simulink model "CSEV"  (R2022b)
settings: Solver=FixedStepDiscrete  StartTime=0.0  StopTime=50000000  FixedStep=1  RelTol=1e-3
libraries: simulink x20
settings Model: Creator=sadamu  LastModifiedBy=程一帆
settings OptimizationCC: DefaultParameterBehavior=Inlined  BufferReuse=off  GlobalBufferReuse=off  ExpressionFolding=off  EnableMemcpy=off  PassReuseOutputArgsAs=Individual arguments  NoFixptDivByZeroProtection=on  EfficientFloat2IntCast=on  OptimizeDataStoreBuffers=off  BusAssignmentInplaceUpdate=off  OptimizationLevel=level0  EfficientTunableParamExpr=on
settings DebuggingCC: ParameterDowncastMsg=warning  ParameterTunabilityLossMsg=error
settings SFSimCC: MATLABDynamicMemAlloc=off
settings RTWCC: Description=Embedded Coder  SystemTargetFile=ert.tlc  GenCodeOnly=on  TemplateMakefile=ert_default_tmf
settings CodeAppCC: ForceParamTrailComments=on  IgnoreCustomStorageClasses=off  OperatorAnnotations=on  SimulinkDataObjDesc=on  SFDataObjDesc=on  InsertBlockDesc=on
settings ERTTargetCC: TargetLangStandard=C99 (ISO)  GenerateSampleERTMain=on  CodeInterfacePackaging=Reusable function  InlinedParameterPlacement=NonHierarchical  ERTCustomFileTemplate=example_file_process.tlc
settings ConfigComp: CovMetricSettings=dcmwe  DVMaxProcessTime=3600  DVTestSuiteOptimization=Auto  DVDetectOutOfBounds=on  DVModelReferenceHarness=on

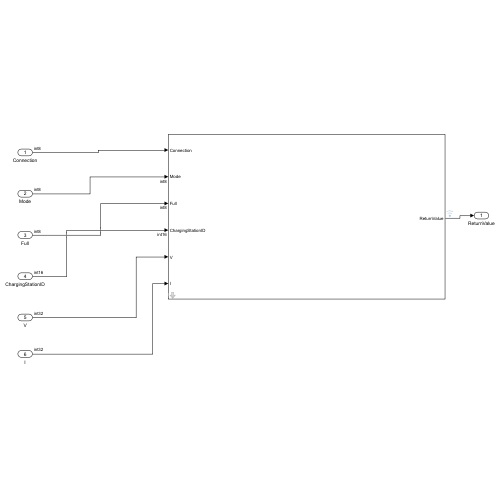
[thumbnail: Simulink's stored preview of the top-level diagram]
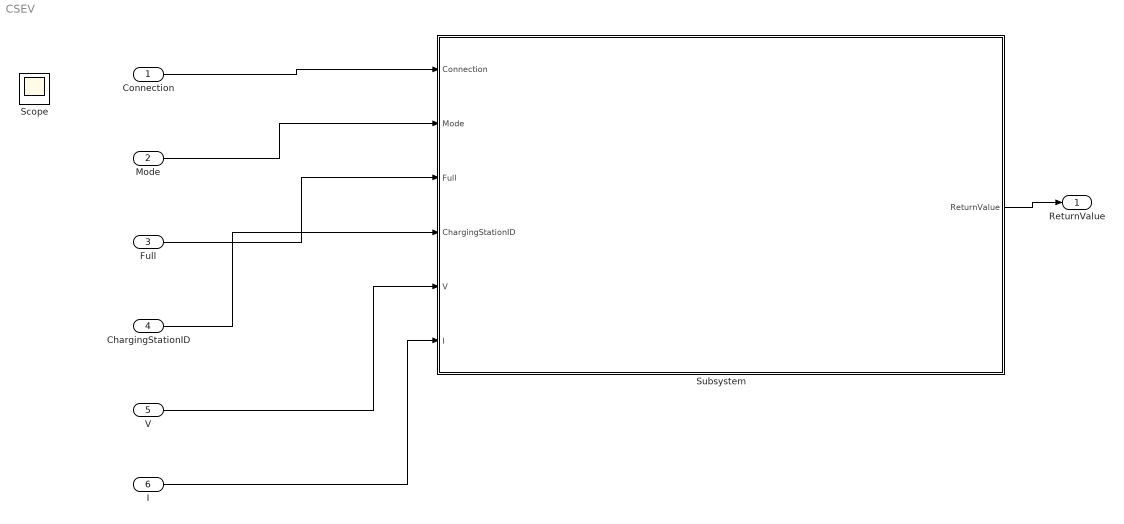
== system CSEV ==
  Connection : Inport  OutDataTypeStr=int8
  Mode : Inport  Port=2  OutDataTypeStr=int8
  Full : Inport  Port=3  OutDataTypeStr=int8
  ChargingStationID : Inport  Port=4  OutDataTypeStr=int16
  V : Inport  Port=5  OutDataTypeStr=int32
  I : Inport  Port=6  OutDataTypeStr=int32
  Subsystem : Subsystem  mask{Len=16}
      mask DialogControl ParameterGroupVar Prompt: 参数
  ReturnValue : Outport
  Scope : Scope
  wires:
  Connection/1 -> Subsystem/1(Connection)
  Mode/1 -> Subsystem/2(Mode)
  Full/1 -> Subsystem/3(Full)
  ChargingStationID/1 -> Subsystem/4(ChargingStationID)
  Subsystem/1(ReturnValue) -> ReturnValue/1
  V/1 -> Subsystem/5(V)
  I/1 -> Subsystem/6(I)

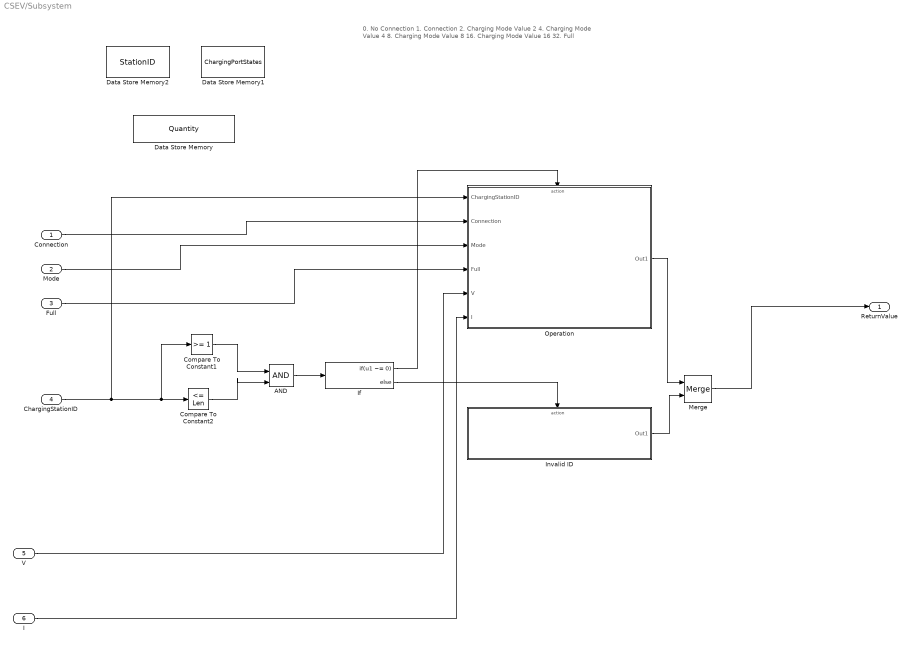
== system CSEV/Subsystem ==
  note: 0. No Connection
      | 1. Connection
      | 2. Charging Mode Value 2
      | 4. Charging Mode Value 4
      | 8. Charging Mode Value 8
      | 16. Charging Mode Value 16
      | 32. Full
  Connection : Inport
  Mode : Inport  Port=2  OutDataTypeStr=int8
  Full : Inport  Port=3  OutDataTypeStr=int8
  ChargingStationID : Inport  Port=4  OutDataTypeStr=int16
  V : Inport  Port=5
  I : Inport  Port=6
  AND : Logic  IconShape=distinctive  AllPortsSameDT=off  OutDataTypeStr=boolean
  Compare To Constant1 : simulink/Logic and Bit Operations/Compare To Constant  relop=>=  const=1  OutDataTypeStr=boolean
  Compare To Constant2 : simulink/Logic and Bit Operations/Compare To Constant  relop=<=  const=Len  OutDataTypeStr=boolean
  Data Store Memory : DataStoreMemory  DataStoreName=Quantity  WriteAfterWriteMsg=warning  ShowAdditionalParam=off  OutDataTypeStr=int64
  Data Store Memory1 : DataStoreMemory  DataStoreName=ChargingPortStates  WriteAfterWriteMsg=warning  ShowAdditionalParam=off  OutDataTypeStr=int32  Dimensions=Len
  Data Store Memory2 : DataStoreMemory  DataStoreName=StationID  WriteAfterWriteMsg=warning  ShowAdditionalParam=off  OutDataTypeStr=int32  Dimensions=Len
  If : If  IfExpression=u1 ~= 0
  Invalid ID : Subsystem  TreatAsAtomicUnit=on
  Merge : Merge
  Operation : Subsystem  TreatAsAtomicUnit=on
  ReturnValue : Outport
  wires:
  Connection/1 -> Operation/2(Connection)
  ChargingStationID/1 -> Operation/1(ChargingStationID), Compare To Constant2/1, Compare To Constant1/1
  Compare To Constant1/1 -> AND/1
  Compare To Constant2/1 -> AND/2
  AND/1 -> If/1
  If/2 -> Invalid ID/Action
  Invalid ID/1(Out1) -> Merge/2
  Merge/1 -> ReturnValue/1
  If/1 -> Operation/Action
  Operation/1(Out1) -> Merge/1
  Mode/1 -> Operation/3(Mode)
  Full/1 -> Operation/4(Full)
  V/1 -> Operation/5(V)
  I/1 -> Operation/6(I)

== system CSEV/Subsystem/Invalid ID ==
  Action Port : ActionPort  ActionPortLabel=else
  Constant : Constant  Value=-1  OutDataTypeStr=int32
  Out1 : Outport
  wires:
  Constant/1 -> Out1/1

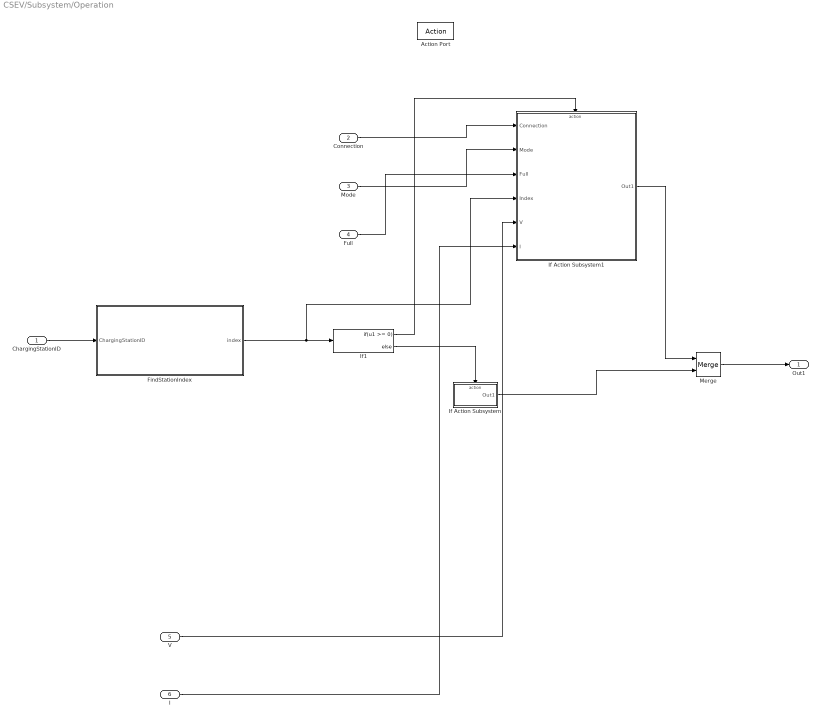
== system CSEV/Subsystem/Operation ==
  ChargingStationID : Inport  OutDataTypeStr=int16
  Connection : Inport  Port=2
  Mode : Inport  Port=3
  Full : Inport  Port=4
  V : Inport  Port=5
  I : Inport  Port=6
  Action Port : ActionPort  ActionPortLabel=if(u1 ~= 0)
  FindStationIndex : Subsystem  TreatAsAtomicUnit=on
  If Action Subsystem : Subsystem  TreatAsAtomicUnit=on
  If Action Subsystem1 : Subsystem  TreatAsAtomicUnit=on
  If1 : If  IfExpression=u1 >= 0
  Merge : Merge
  Out1 : Outport
  wires:
  ChargingStationID/1 -> FindStationIndex/1(ChargingStationID)
  FindStationIndex/1(index) -> If Action Subsystem1/4(Index), If1/1
  If1/2 -> If Action Subsystem/Action
  If1/1 -> If Action Subsystem1/Action
  If Action Subsystem1/1(Out1) -> Merge/1
  If Action Subsystem/1(Out1) -> Merge/2
  Merge/1 -> Out1/1
  Mode/1 -> If Action Subsystem1/2(Mode)
  Connection/1 -> If Action Subsystem1/1(Connection)
  Full/1 -> If Action Subsystem1/3(Full)
  V/1 -> If Action Subsystem1/5(V)
  I/1 -> If Action Subsystem1/6(I)

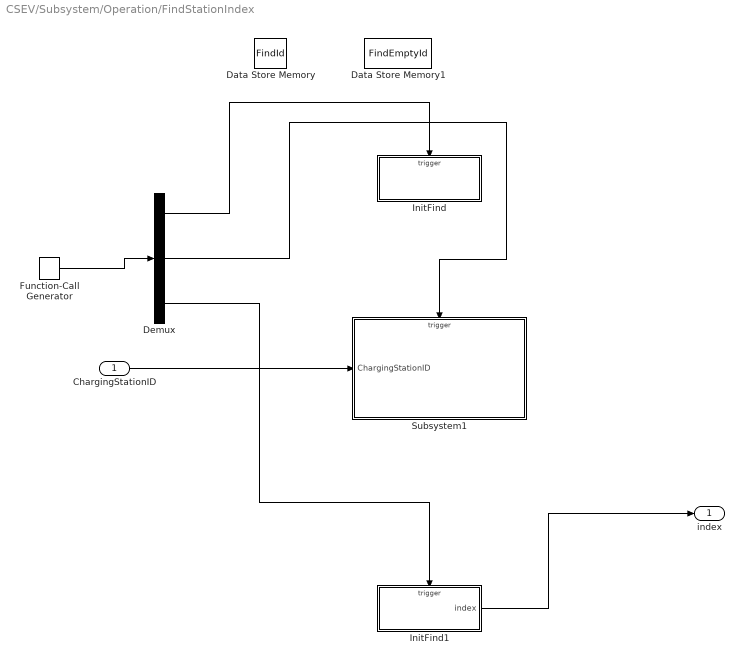
== system CSEV/Subsystem/Operation/FindStationIndex ==
  ChargingStationID : Inport
  Data Store Memory : DataStoreMemory  DataStoreName=FindId  WriteAfterWriteMsg=warning  ShowAdditionalParam=off  OutDataTypeStr=int16
  Data Store Memory1 : DataStoreMemory  DataStoreName=FindEmptyId  WriteAfterWriteMsg=warning  ShowAdditionalParam=off  OutDataTypeStr=int16
  Demux : Demux  Outputs=3
  Function-Call Generator : simulink/Ports & Subsystems/Function-Call Generator  sample_time=1  numberOfIterations=1  DisallowWideOutput=off
  InitFind : Subsystem
  InitFind1 : Subsystem
  Subsystem1 : Subsystem
  index : Outport
  wires:
  Function-Call Generator/1 -> Demux/1
  Demux/1 -> InitFind/Trigger
  Demux/2 -> Subsystem1/Trigger
  ChargingStationID/1 -> Subsystem1/1(ChargingStationID)
  InitFind1/1(index) -> index/1
  Demux/3 -> InitFind1/Trigger

== system CSEV/Subsystem/Operation/If Action Subsystem ==
  Action Port : ActionPort  ActionPortLabel=else
  Constant : Constant  Value=-2  OutDataTypeStr=int32
  Out1 : Outport
  wires:
  Constant/1 -> Out1/1

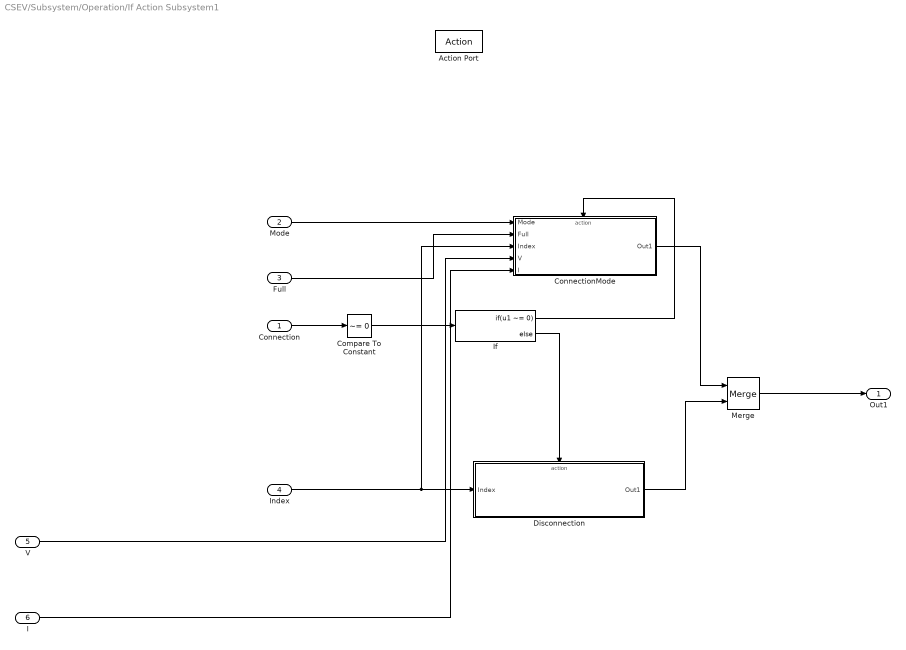
== system CSEV/Subsystem/Operation/If Action Subsystem1 ==
  Connection : Inport
  Mode : Inport  Port=2
  Full : Inport  Port=3
  Index : Inport  Port=4  OutDataTypeStr=int16
  V : Inport  Port=5
  I : Inport  Port=6
  Action Port : ActionPort  ActionPortLabel=if(u1 >= 0)
  Compare To Constant : simulink/Logic and Bit Operations/Compare To Constant  relop=~=  const=0  OutDataTypeStr=boolean
  ConnectionMode : Subsystem  TreatAsAtomicUnit=on
  Disconnection : Subsystem  TreatAsAtomicUnit=on
  If : If  IfExpression=u1 ~= 0
  Merge : Merge
  Out1 : Outport
  wires:
  Mode/1 -> ConnectionMode/1(Mode)
  Index/1 -> ConnectionMode/3(Index), Disconnection/1(Index)
  Compare To Constant/1 -> If/1
  If/2 -> Disconnection/Action
  Full/1 -> ConnectionMode/2(Full)
  Connection/1 -> Compare To Constant/1
  If/1 -> ConnectionMode/Action
  ConnectionMode/1(Out1) -> Merge/1
  Disconnection/1(Out1) -> Merge/2
  Merge/1 -> Out1/1
  V/1 -> ConnectionMode/4(V)
  I/1 -> ConnectionMode/5(I)

== system CSEV/Subsystem/Operation/FindStationIndex/InitFind ==
  function : TriggerPort  TriggerType=function-call  VariantControl=Variant
  Constant : Constant  Value=-1  OutDataTypeStr=int16
  Constant1 : Constant  Value=-1  OutDataTypeStr=int16
  Data Store Write : DataStoreWrite  DataStoreName=FindEmptyId  IndexOptions=Index vector (dialog)  Indices=1  OutputSizes=1
  Data Store Write1 : DataStoreWrite  DataStoreName=FindId  IndexOptions=Index vector (dialog)  Indices=1  OutputSizes=1
  wires:
  Constant/1 -> Data Store Write1/1
  Constant1/1 -> Data Store Write/1

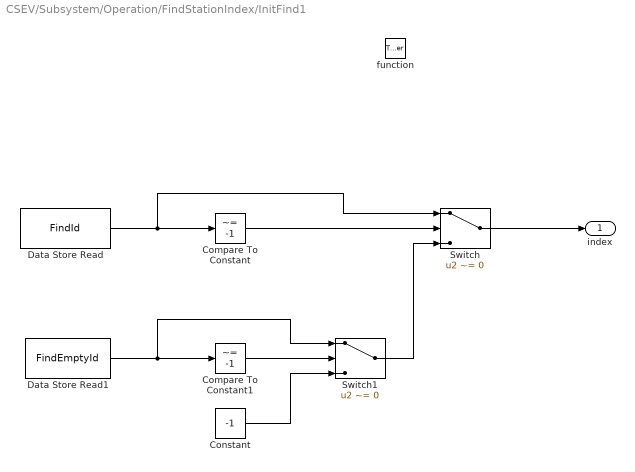
== system CSEV/Subsystem/Operation/FindStationIndex/InitFind1 ==
  function : TriggerPort  TriggerType=function-call  VariantControl=Variant
  Compare To Constant : simulink/Logic and Bit Operations/Compare To Constant  relop=~=  const=-1  OutDataTypeStr=boolean
  Compare To Constant1 : simulink/Logic and Bit Operations/Compare To Constant  relop=~=  const=-1  OutDataTypeStr=boolean
  Constant : Constant  Value=-1  OutDataTypeStr=int16
  Data Store Read : DataStoreRead  DataStoreName=FindId  IndexOptions=Index vector (dialog)  Indices=1  OutputSizes=1
  Data Store Read1 : DataStoreRead  DataStoreName=FindEmptyId  IndexOptions=Index vector (dialog)  Indices=1  OutputSizes=1
  Switch : Switch  Criteria=u2 ~= 0  SaturateOnIntegerOverflow=off  InputSameDT=off
  Switch1 : Switch  Criteria=u2 ~= 0  SaturateOnIntegerOverflow=off  InputSameDT=off
  index : Outport
  wires:
  Data Store Read/1 -> Switch/1, Compare To Constant/1
  Compare To Constant/1 -> Switch/2
  Data Store Read1/1 -> Switch1/1, Compare To Constant1/1
  Compare To Constant1/1 -> Switch1/2
  Switch1/1 -> Switch/3
  Constant/1 -> Switch1/3
  Switch/1 -> index/1

== system CSEV/Subsystem/Operation/FindStationIndex/Subsystem1 ==
  ChargingStationID : Inport
  function : TriggerPort  TriggerType=function-call  VariantControl=Variant
  Subsystem : Subsystem
  wires:
  ChargingStationID/1 -> Subsystem/1(ChargingStationID)

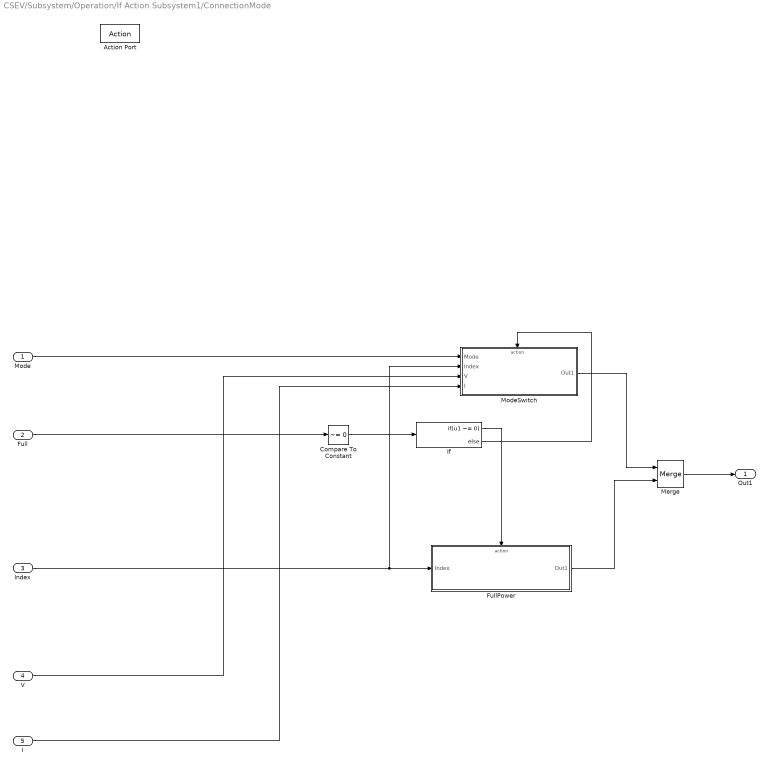
== system CSEV/Subsystem/Operation/If Action Subsystem1/ConnectionMode ==
  Mode : Inport
  Full : Inport  Port=2
  Index : Inport  Port=3  OutDataTypeStr=int16
  V : Inport  Port=4
  I : Inport  Port=5
  Action Port : ActionPort  ActionPortLabel=if(u1 ~= 0)
  Compare To Constant : simulink/Logic and Bit Operations/Compare To Constant  relop=~=  const=0  OutDataTypeStr=boolean
  FullPower : Subsystem  TreatAsAtomicUnit=on
  If : If  IfExpression=u1 ~= 0
  Merge : Merge
  ModeSwitch : Subsystem  TreatAsAtomicUnit=on
  Out1 : Outport
  wires:
  Index/1 -> ModeSwitch/2(Index), FullPower/1(Index)
  Mode/1 -> ModeSwitch/1(Mode)
  Compare To Constant/1 -> If/1
  If/2 -> ModeSwitch/Action
  Full/1 -> Compare To Constant/1
  If/1 -> FullPower/Action
  ModeSwitch/1(Out1) -> Merge/1
  FullPower/1(Out1) -> Merge/2
  Merge/1 -> Out1/1
  V/1 -> ModeSwitch/3(V)
  I/1 -> ModeSwitch/4(I)

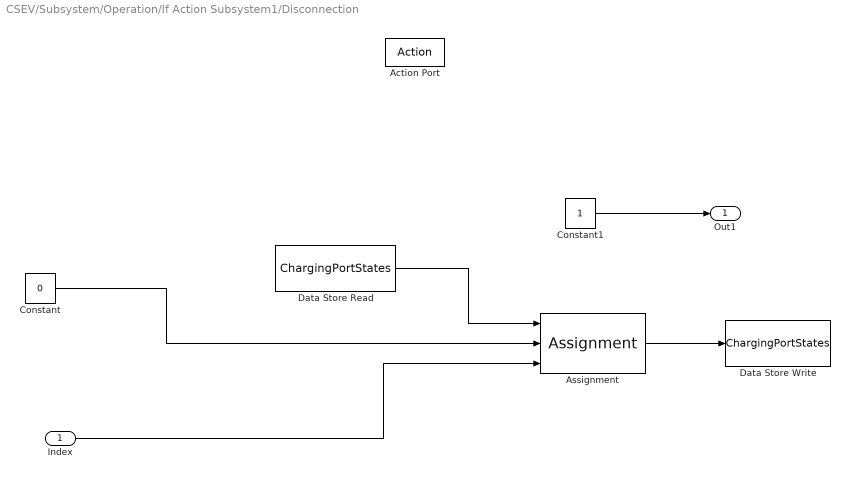
== system CSEV/Subsystem/Operation/If Action Subsystem1/Disconnection ==
  Index : Inport
  Action Port : ActionPort  ActionPortLabel=else
  Assignment : Assignment  IndexMode=Zero-based  DiagnosticForDimensions=Warning  IndexOptions=Index vector (port)  Indices=1  OutputSizes=1
  Constant : Constant  Value=0  OutDataTypeStr=int32
  Constant1 : Constant  OutDataTypeStr=int32
  Data Store Read : DataStoreRead  DataStoreName=ChargingPortStates  IndexOptions=Index vector (dialog)  Indices=1  OutputSizes=1
  Data Store Write : DataStoreWrite  DataStoreName=ChargingPortStates  IndexOptions=Index vector (dialog)  Indices=1  OutputSizes=1
  Out1 : Outport
  wires:
  Data Store Read/1 -> Assignment/1
  Assignment/1 -> Data Store Write/1
  Index/1 -> Assignment/3
  Constant/1 -> Assignment/2
  Constant1/1 -> Out1/1

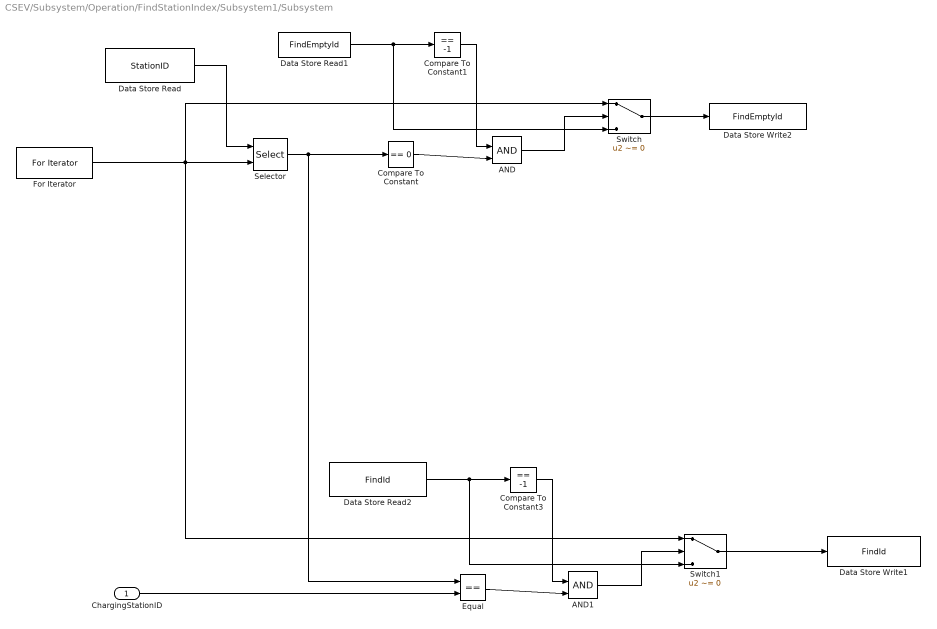
== system CSEV/Subsystem/Operation/FindStationIndex/Subsystem1/Subsystem ==
  ChargingStationID : Inport
  AND : Logic  IconShape=distinctive  AllPortsSameDT=off  OutDataTypeStr=boolean
  AND1 : Logic  IconShape=distinctive  AllPortsSameDT=off  OutDataTypeStr=boolean
  Compare To Constant : simulink/Logic and Bit Operations/Compare To Constant  relop===  const=0  OutDataTypeStr=boolean
  Compare To Constant1 : simulink/Logic and Bit Operations/Compare To Constant  relop===  const=-1  OutDataTypeStr=boolean
  Compare To Constant3 : simulink/Logic and Bit Operations/Compare To Constant  relop===  const=-1  OutDataTypeStr=boolean
  Data Store Read : DataStoreRead  DataStoreName=StationID  IndexOptions=Index vector (dialog)  Indices=1  OutputSizes=1
  Data Store Read1 : DataStoreRead  DataStoreName=FindEmptyId  IndexOptions=Index vector (dialog)  Indices=1  OutputSizes=1
  Data Store Read2 : DataStoreRead  DataStoreName=FindId  IndexOptions=Index vector (dialog)  Indices=1  OutputSizes=1
  Data Store Write1 : DataStoreWrite  DataStoreName=FindId  IndexOptions=Index vector (dialog)  Indices=1  OutputSizes=1
  Data Store Write2 : DataStoreWrite  DataStoreName=FindEmptyId  IndexOptions=Index vector (dialog)  Indices=1  OutputSizes=1
  Equal : RelationalOperator  Operator===  OutDataTypeStr=boolean  RndMeth=Simplest  InputSameDT=off
  For Iterator : ForIterator  IterationLimit=Len  IndexMode=Zero-based  IterationVariableDataType=int16
  Selector : Selector  IndexMode=Zero-based  InputPortWidth=Len  IndexOptions=Index vector (port)  Indices=[1 3]  OutputSizes=1
  Switch : Switch  Criteria=u2 ~= 0  SaturateOnIntegerOverflow=off  InputSameDT=off
  Switch1 : Switch  Criteria=u2 ~= 0  SaturateOnIntegerOverflow=off  InputSameDT=off
  wires:
  Data Store Read/1 -> Selector/1
  Selector/1 -> Equal/1, Compare To Constant/1
  Compare To Constant/1 -> AND/2
  Data Store Read1/1 -> Switch/3, Compare To Constant1/1
  Compare To Constant1/1 -> AND/1
  AND/1 -> Switch/2
  Switch/1 -> Data Store Write2/1
  Equal/1 -> AND1/2
  AND1/1 -> Switch1/2
  Compare To Constant3/1 -> AND1/1
  Data Store Read2/1 -> Switch1/3, Compare To Constant3/1
  Switch1/1 -> Data Store Write1/1
  ChargingStationID/1 -> Equal/2
  For Iterator/1 -> Switch1/1, Switch/1, Selector/2

== system CSEV/Subsystem/Operation/If Action Subsystem1/ConnectionMode/FullPower ==
  Index : Inport
  Action Port : ActionPort  ActionPortLabel=if(u1 ~= 0)
  Assignment : Assignment  IndexMode=Zero-based  DiagnosticForDimensions=Warning  IndexOptions=Index vector (port)  Indices=1  OutputSizes=1
  Constant : Constant  Value=32  OutDataTypeStr=int32
  Constant1 : Constant  OutDataTypeStr=int32
  Data Store Read : DataStoreRead  DataStoreName=ChargingPortStates  IndexOptions=Index vector (dialog)  Indices=1  OutputSizes=1
  Data Store Write : DataStoreWrite  DataStoreName=ChargingPortStates  IndexOptions=Index vector (dialog)  Indices=1  OutputSizes=1
  Out1 : Outport
  wires:
  Data Store Read/1 -> Assignment/1
  Assignment/1 -> Data Store Write/1
  Index/1 -> Assignment/3
  Constant/1 -> Assignment/2
  Constant1/1 -> Out1/1

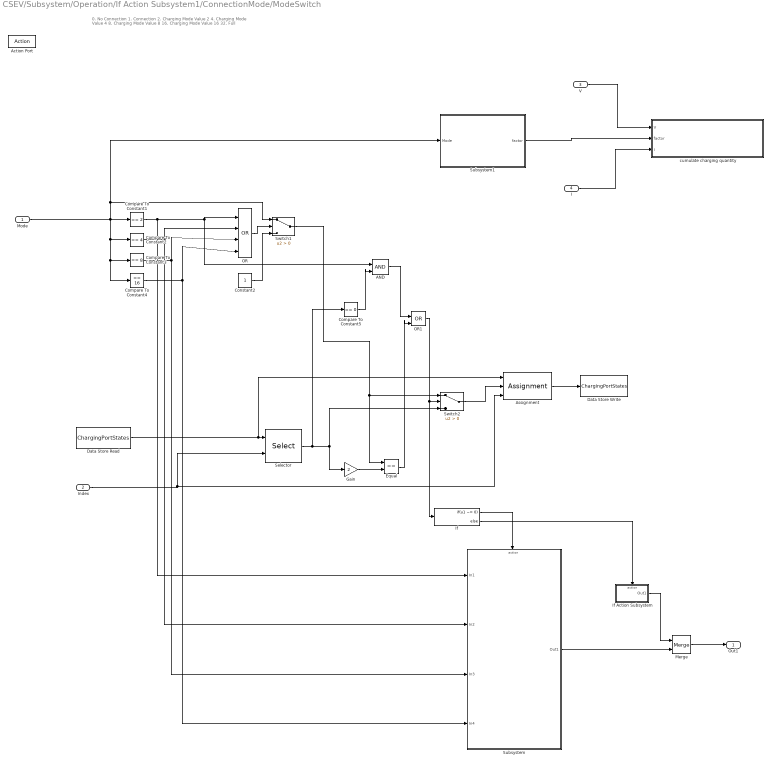
== system CSEV/Subsystem/Operation/If Action Subsystem1/ConnectionMode/ModeSwitch ==
  note: 0. No Connection
      | 1. Connection
      | 2. Charging Mode Value 2
      | 4. Charging Mode Value 4
      | 8. Charging Mode Value 8
      | 16. Charging Mode Value 16
      | 32. Full
  Mode : Inport
  Index : Inport  Port=2  OutDataTypeStr=int16
  V : Inport  Port=3
  I : Inport  Port=4
  Action Port : ActionPort  ActionPortLabel=else
  AND : Logic  IconShape=distinctive  AllPortsSameDT=off  OutDataTypeStr=boolean
  Assignment : Assignment  IndexMode=Zero-based  DiagnosticForDimensions=Warning  IndexOptions=Index vector (port)  Indices=1  OutputSizes=1
  Compare To Constant1 : simulink/Logic and Bit Operations/Compare To Constant  relop===  const=2  OutDataTypeStr=boolean
  Compare To Constant2 : simulink/Logic and Bit Operations/Compare To Constant  relop===  const=4  OutDataTypeStr=boolean
  Compare To Constant3 : simulink/Logic and Bit Operations/Compare To Constant  relop===  const=8  OutDataTypeStr=boolean
  Compare To Constant4 : simulink/Logic and Bit Operations/Compare To Constant  relop===  const=16  OutDataTypeStr=boolean
  Compare To Constant5 : simulink/Logic and Bit Operations/Compare To Constant  relop===  const=0  OutDataTypeStr=boolean
  Constant2 : Constant  OutDataTypeStr=int32
  Data Store Read : DataStoreRead  DataStoreName=ChargingPortStates  IndexOptions=Index vector (dialog)  Indices=1  OutputSizes=1
  Data Store Write : DataStoreWrite  DataStoreName=ChargingPortStates  IndexOptions=Index vector (dialog)  Indices=1  OutputSizes=1
  Equal : RelationalOperator  Operator===  OutDataTypeStr=boolean  RndMeth=Simplest  InputSameDT=off
  Gain : Gain  Gain=2  OutDataTypeStr=int32
  If : If  IfExpression=u1 ~= 0
  If Action Subsystem : Subsystem  TreatAsAtomicUnit=on
  Merge : Merge
  OR : Logic  Operator=OR  Inputs=4  IconShape=distinctive  AllPortsSameDT=off  OutDataTypeStr=boolean
  OR1 : Logic  Operator=OR  IconShape=distinctive  AllPortsSameDT=off  OutDataTypeStr=boolean
  Selector : Selector  IndexMode=Zero-based  InputPortWidth=Len  IndexOptions=Index vector (port)  Indices=[1 3]  OutputSizes=1
  Subsystem : Subsystem
  Subsystem1 : Subsystem
  Switch1 : Switch  Criteria=u2 > Threshold  SaturateOnIntegerOverflow=off  InputSameDT=off
  Switch2 : Switch  Criteria=u2 > Threshold  SaturateOnIntegerOverflow=off  InputSameDT=off
  cumulate charging quantity : Subsystem
  Out1 : Outport
  wires:
  Switch1/1 -> Equal/1, Switch2/1
  Data Store Read/1 -> Assignment/1, Selector/1
  OR/1 -> Switch1/2
  Compare To Constant3/1 -> Subsystem/3(In3), OR/3
  Compare To Constant4/1 -> Subsystem/4(In4), OR/4
  Compare To Constant1/1 -> Subsystem/1(In1), AND/1, OR/1
  Compare To Constant2/1 -> Subsystem/2(In2), OR/2
  Mode/1 -> Subsystem1/1(Mode), Switch1/1, Compare To Constant1/1, Compare To Constant4/1, Compare To Constant3/1, Compare To Constant2/1
  Constant2/1 -> Switch1/3
  Assignment/1 -> Data Store Write/1
  Index/1 -> Selector/2, Assignment/3
  Selector/1 -> Compare To Constant5/1, Gain/1, Switch2/3
  Switch2/1 -> Assignment/2
  If Action Subsystem/1(Out1) -> Merge/1
  Subsystem/1(Out1) -> Merge/2
  Merge/1 -> Out1/1
  Gain/1 -> Equal/2
  If/1 -> Subsystem/Action
  If/2 -> If Action Subsystem/Action
  Compare To Constant5/1 -> AND/2
  AND/1 -> OR1/1
  Equal/1 -> OR1/2
  OR1/1 -> If/1, Switch2/2
  V/1 -> cumulate charging quantity/1(V)
  I/1 -> cumulate charging quantity/3(I)
  Subsystem1/1(factor) -> cumulate charging quantity/2(factor)

== system CSEV/Subsystem/Operation/If Action Subsystem1/ConnectionMode/ModeSwitch/If Action Subsystem ==
  Action Port : ActionPort  ActionPortLabel=else
  Constant2 : Constant  Value=32  OutDataTypeStr=int32
  Out1 : Outport
  wires:
  Constant2/1 -> Out1/1

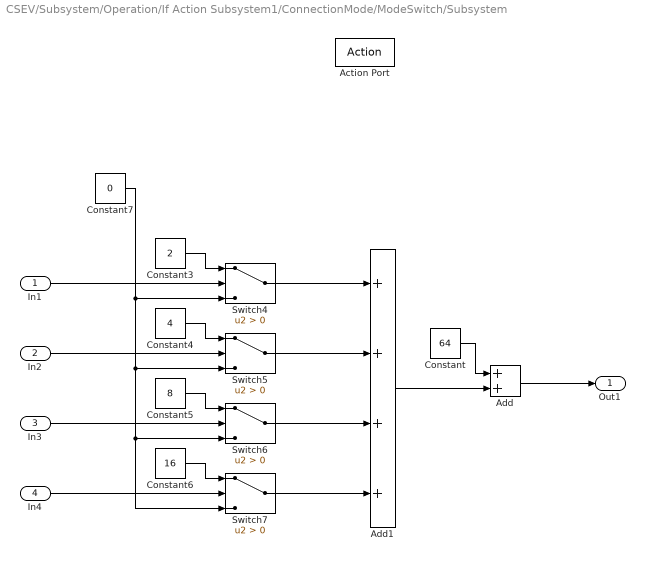
== system CSEV/Subsystem/Operation/If Action Subsystem1/ConnectionMode/ModeSwitch/Subsystem ==
  In1 : Inport
  In2 : Inport  Port=2
  In3 : Inport  Port=3
  In4 : Inport  Port=4
  Action Port : ActionPort  ActionPortLabel=if(u1 ~= 0)
  Add : Sum
  Add1 : Sum  Inputs=++++
  Constant : Constant  Value=64  OutDataTypeStr=int32
  Constant3 : Constant  Value=2  OutDataTypeStr=int32
  Constant4 : Constant  Value=4  OutDataTypeStr=int32
  Constant5 : Constant  Value=8  OutDataTypeStr=int32
  Constant6 : Constant  Value=16  OutDataTypeStr=int32
  Constant7 : Constant  Value=0  OutDataTypeStr=int32
  Switch{4..7} (4 alike) : Switch  Criteria=u2 > Threshold  SaturateOnIntegerOverflow=off  InputSameDT=off
  Out1 : Outport
  wires:
  Constant6/1 -> Switch7/1
  In1/1 -> Switch4/2
  Switch5/1 -> Add1/2
  Add1/1 -> Add/2
  Add/1 -> Out1/1
  Constant5/1 -> Switch6/1
  Constant4/1 -> Switch5/1
  Switch6/1 -> Add1/3
  Constant3/1 -> Switch4/1
  Switch7/1 -> Add1/4
  Switch4/1 -> Add1/1
  Constant7/1 -> Switch7/3, Switch6/3, Switch5/3, Switch4/3
  In4/1 -> Switch7/2
  Constant/1 -> Add/1
  In3/1 -> Switch6/2
  In2/1 -> Switch5/2

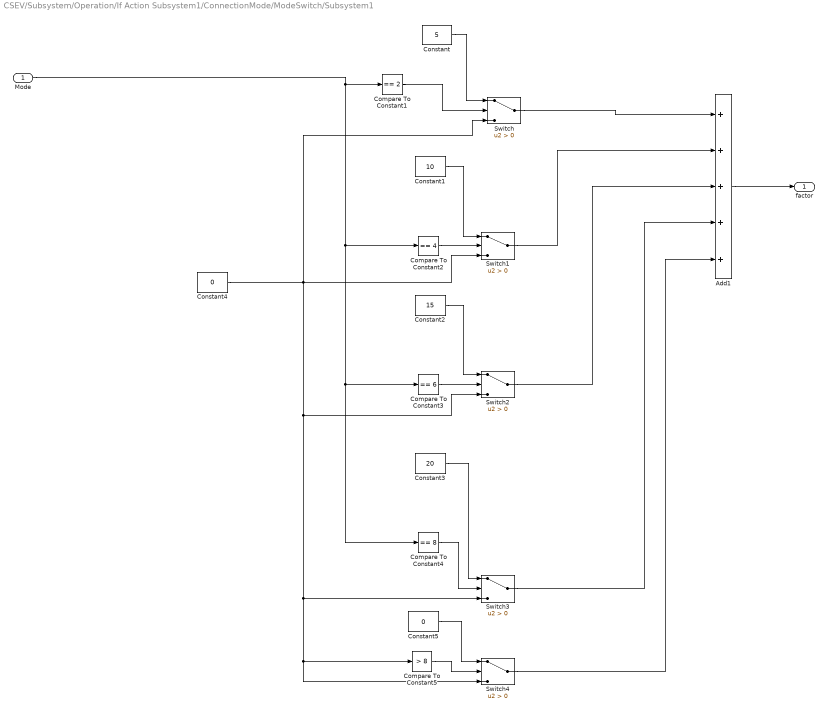
== system CSEV/Subsystem/Operation/If Action Subsystem1/ConnectionMode/ModeSwitch/Subsystem1 ==
  Mode : Inport
  Add1 : Sum  Inputs=+++++
  Compare To Constant1 : simulink/Logic and Bit Operations/Compare To Constant  relop===  const=2  OutDataTypeStr=boolean
  Compare To Constant2 : simulink/Logic and Bit Operations/Compare To Constant  relop===  const=4  OutDataTypeStr=boolean
  Compare To Constant3 : simulink/Logic and Bit Operations/Compare To Constant  relop===  const=6  OutDataTypeStr=boolean
  Compare To Constant4 : simulink/Logic and Bit Operations/Compare To Constant  relop===  const=8  OutDataTypeStr=boolean
  Compare To Constant5 : simulink/Logic and Bit Operations/Compare To Constant  relop=>  const=8  OutDataTypeStr=boolean
  Constant : Constant  Value=5  OutDataTypeStr=int32
  Constant1 : Constant  Value=10  OutDataTypeStr=int32
  Constant2 : Constant  Value=15  OutDataTypeStr=int32
  Constant3 : Constant  Value=20  OutDataTypeStr=int32
  Constant4 : Constant  Value=0  OutDataTypeStr=int32
  Constant5 : Constant  Value=0  OutDataTypeStr=int32
  Switch{,1..4} (5 alike) : Switch  Criteria=u2 > Threshold  SaturateOnIntegerOverflow=off  InputSameDT=off
  factor : Outport
  wires:
  Compare To Constant1/1 -> Switch/2
  Constant/1 -> Switch/1
  Switch/1 -> Add1/1
  Constant1/1 -> Switch1/1
  Compare To Constant2/1 -> Switch1/2
  Switch1/1 -> Add1/2
  Constant2/1 -> Switch2/1
  Compare To Constant3/1 -> Switch2/2
  Switch2/1 -> Add1/3
  Switch3/1 -> Add1/4
  Mode/1 -> Compare To Constant2/1, Compare To Constant3/1, Compare To Constant4/1, Compare To Constant1/1
  Compare To Constant4/1 -> Switch3/2
  Constant3/1 -> Switch3/1
  Constant4/1 -> Switch/3, Switch1/3, Switch2/3, Switch3/3, Compare To Constant5/1, Switch4/3
  Compare To Constant5/1 -> Switch4/2
  Constant5/1 -> Switch4/1
  Switch4/1 -> Add1/5
  Add1/1 -> factor/1

== system CSEV/Subsystem/Operation/If Action Subsystem1/ConnectionMode/ModeSwitch/cumulate charging quantity ==
  V : Inport
  factor : Inport  Port=2
  I : Inport  Port=3
  Data Store Read1 : DataStoreRead  DataStoreName=Quantity  IndexOptions=Index vector (dialog)  Indices=1  OutputSizes=1
  Data Store Write1 : DataStoreWrite  DataStoreName=Quantity  IndexOptions=Index vector (dialog)  Indices=1  OutputSizes=1
  Product : Product  OutDataTypeStr=int32
  Product1 : Product  OutDataTypeStr=int32
  Sum : Sum  Inputs=|++  OutDataTypeStr=int64
  wires:
  Product/1 -> Product1/1
  V/1 -> Product/1
  Sum/1 -> Data Store Write1/1
  factor/1 -> Product1/2
  Data Store Read1/1 -> Sum/2
  I/1 -> Product/2
  Product1/1 -> Sum/1
